simulink model "test"  (R2019b)
settings: Solver=ode45  StartTime=0  StopTime=600  FixedStep=1  MaxStep=1  RelTol=1e-3  EnableMultiTasking=on
values from neighbouring files (symbols this model uses):
  hardware = load_hardware(hardwareN,hardware)    [Simulator.m]
  scenario = Lscenario(scen)    [Simulator.m]    (also in init.m)
  struttura = Lst(ind)    [Simulator.m]    (also in init.m)
undefined symbols (not defined in the file or in its folder): ctrller
settings Model: Creator=Marc Breton  LastModifiedBy=CSLAB
settings SolverCC: InitialStep=0.1
settings DataIOCC: ExternalInput=[t,u]  SaveFormat=Array  SignalLoggingSaveFormat=ModelDataLogs  SaveOutput=off  SignalLogging=off  SaveTime=off  ReturnWorkspaceOutputs=off
settings OptimizationCC: ExpressionDepthLimit=2147483647  InitFltsAndDblsToZero=on  LifeSpan=inf
settings DebuggingCC: SaveWithParameterizedLinksMsg=none  UnderspecifiedInitializationDetection=Classic  MergeDetectMultiDrivingBlocksExec=none  SignalResolutionControl=TryResolveAllWithWarning  SolverPrmCheckMsg=warning  InheritedTsInSrcMsg=none  MultiTaskDSMMsg=warning  MultiTaskCondExecSysMsg=none  FcnCallInpInsideContextMsg=warning  StateNameClashWarn=warning  SFUnexpectedBacktrackingDiag=warning  SFNoUnconditionalDefaultTransitionDiag=warning  SFExecutionAtInitializationDiag=none  ArithmeticOperatorsInVariantConditions=warning
settings HardwareCC: ProdBitPerPointer=32  ProdBitPerSizeT=32  ProdBitPerPtrDiffT=32  ProdLargestAtomicFloat=None  ProdIntDivRoundTo=Undefined  ProdEndianess=Unspecified  ProdWordSize=32  ProdHWDeviceType=32-bit Generic
settings ModelReferenceCC: PropagateSignalLabelsOutOfModel=off
settings SFSimCC: SimUseLocalCustomCode=off  CustomCodeUndefinedFunction=UseInterfaceOnly
settings RTWCC: RTWUseLocalCustomCode=off
settings CodeAppCC: StateflowObjectComments=on
settings GRTTargetCC: TargetFcnLib=ansi_tfl_tmw.mat  TargetLangStandard=C89/C90 (ANSI)  GeneratePreprocessorConditionals=Disable all  CombineOutputUpdateFcns=off  GRTInterface=on
settings ConfigComp: CovMetricSettings=dw  CovHtmlReporting=on  CovSaveCumulativeToWorkspaceVar=on  CovSaveSingleToWorkspaceVar=on  CovExternalEMLEnable=off

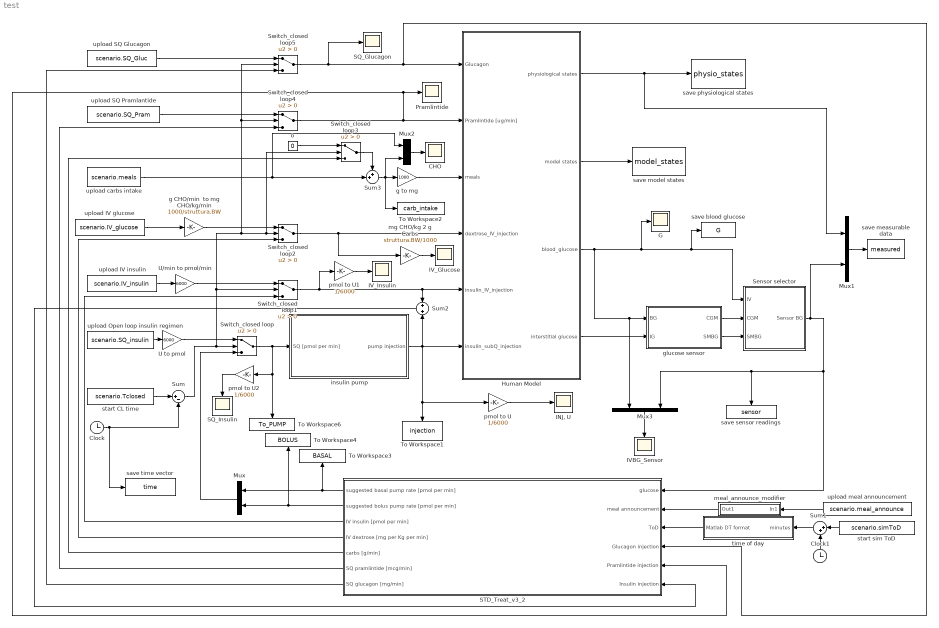
== system test ==
  CHO : Scope
  Clock : Clock
  Clock1 : Clock
  G : Scope
  Human Model : Subsystem
  "INJ, U" : Scope
  IVBG_Sensor : Scope
  IV_Glucose : Scope
  IV_Insulin : Scope
  Mux{,1..3} (4 alike) : Mux  Inputs=2
  Pramlintide : Scope
  SQ_Glucagon : Scope
  SQ_Insulin : Scope
  STD_Treat_v3_2 : Subsystem
  Sensor selector : Subsystem
  Sum : Sum  Inputs=|+-
  Sum1 : Sum  Inputs=|++
  Sum2 : Sum  Inputs=+|+
  Sum3 : Sum  Inputs=++|
  Switch_closed loop{,1..5} (6 alike) : Switch  Criteria=u2 > Threshold
  To Workspace1 : ToWorkspace  VariableName=injection  SaveFormat=Structure  SampleTime=-1
  To Workspace2 : ToWorkspace  VariableName=carb_intake  SaveFormat=Structure  SampleTime=-1
  To Workspace3 : ToWorkspace  VariableName=BASAL  SaveFormat=Structure  SampleTime=-1
  To Workspace4 : ToWorkspace  VariableName=BOLUS  SaveFormat=Structure  SampleTime=-1
  To Workspace6 : ToWorkspace  VariableName=To_PUMP  SaveFormat=Structure  SampleTime=-1
  U to pmol : Gain  Gain=6000
  U/min to pmol/min : Gain  Gain=6000
  g CHO/min  to mg CHO/kg/min : Gain  Gain=1000/struttura.BW
  g to mg : Gain  Gain=1000
  glucose sensor : Subsystem
  insulin pump : Subsystem
  meal_announce_modifier : Subsystem
  mg CHO/kg 2 g Carbs : Gain  Gain=struttura.BW/1000
  o : Constant  Value=0
  pmol to U : Gain  Gain=1/6000
  pmol to U1 : Gain  Gain=1/6000
  pmol to U2 : Gain  Gain=1/6000
  save blood glucose : ToWorkspace  VariableName=G  SaveFormat=Structure  SampleTime=-1
  save measurable data : ToWorkspace  VariableName=measured  SaveFormat=Structure  SampleTime=-1
  save model states : ToWorkspace  VariableName=model_states  SaveFormat=Structure With Time  SampleTime=-1
  save physiological states : ToWorkspace  VariableName=physio_states  SaveFormat=Structure With Time  SampleTime=-1
  save sensor readings : ToWorkspace  VariableName=sensor  SaveFormat=Structure  SampleTime=-1
  save time vector : ToWorkspace  VariableName=time  SaveFormat=Structure  SampleTime=-1
  start CL time : Constant  Value=scenario.Tclosed
  start sim ToD : Constant  Value=scenario.simToD
  time of day : Subsystem
  "upload IV glucose " : FromWorkspace  VariableName=scenario.IV_glucose  SampleTime=0
  upload IV insulin : FromWorkspace  VariableName=scenario.IV_insulin  SampleTime=0
  upload Open loop insulin regimen : FromWorkspace  VariableName=scenario.SQ_insulin  SampleTime=0
  upload SQ Glucagon : FromWorkspace  VariableName=scenario.SQ_Gluc  SampleTime=0
  upload SQ Pramlantide : FromWorkspace  VariableName=scenario.SQ_Pram  SampleTime=0
  upload carbs intake : FromWorkspace  VariableName=scenario.meals  SampleTime=0
  upload meal announcement : FromWorkspace  VariableName=scenario.meal_announce  SampleTime=0
  wires:
  Clock/1 -> Sum/2, save time vector/1
  upload carbs intake/1 -> Mux2/1, Sum3/2
  upload Open loop insulin regimen/1 -> U to pmol/1
  start CL time/1 -> Sum/1
  Sum/1 -> Switch_closed loop/2, Switch_closed loop1/2, Switch_closed loop2/2, Switch_closed loop3/2, Switch_closed loop4/2, Switch_closed loop5/2
  U to pmol/1 -> Switch_closed loop/1
  insulin pump/1(pump injection) -> Human Model/6(insulin_subQ_injection), Sum2/2, To Workspace1/1, pmol to U/1
  Switch_closed loop/1 -> To Workspace6/1, pmol to U2/1, insulin pump/1(SQ [pmol per min])
  STD_Treat_v3_2/1(suggested basal pump rate [pmol per min]) -> Mux/1, To Workspace3/1
  Mux/1 -> Switch_closed loop/3
  start sim ToD/1 -> Sum1/1
  Sum1/1 -> time of day/1(minutes)
  Human Model/1(physiological states) -> save physiological states/1, Mux1/1
  Human Model/2(model states) -> save model states/1
  Human Model/4(interstitial glucose) -> glucose sensor/2(IG)
  "upload IV glucose "/1 -> g CHO/min  to mg CHO/kg/min/1
  upload IV insulin/1 -> U/min to pmol/min/1
  glucose sensor/1(CGM) -> Sensor selector/2(CGM)
  Sensor selector/1(Sensor BG) -> Mux1/2, Mux3/2, save sensor readings/1, STD_Treat_v3_2/1(glucose)
  Sum2/1 -> STD_Treat_v3_2/6(Insulin injection)
  Mux1/1 -> save measurable data/1
  U/min to pmol/min/1 -> Switch_closed loop1/1
  g CHO/min  to mg CHO/kg/min/1 -> Switch_closed loop2/1
  Switch_closed loop1/1 -> Sum2/1, Human Model/5(insulin_IV_injection), pmol to U1/1
  STD_Treat_v3_2/3(IV insulin [pmol per min]) -> Switch_closed loop1/3
  Sum3/1 -> g to mg/1, To Workspace2/1, Mux2/2
  Switch_closed loop3/1 -> Sum3/1
  o/1 -> Switch_closed loop3/1
  glucose sensor/2(SMBG) -> Sensor selector/3(SMBG)
  Clock1/1 -> Sum1/2
  STD_Treat_v3_2/2(suggested bolus pump rate [pmol per min]) -> Mux/2, To Workspace4/1
  STD_Treat_v3_2/4(IV dextrose [mg per Kg per min]) -> Switch_closed loop2/3
  STD_Treat_v3_2/5(carbs [g/min]) -> Switch_closed loop3/3
  time of day/1(Matlab DT format) -> STD_Treat_v3_2/3(ToD)
  pmol to U/1 -> "INJ, U"/1
  upload SQ Pramlantide/1 -> Switch_closed loop4/1
  STD_Treat_v3_2/6(SQ pramlintide [mcg/min]) -> Switch_closed loop4/3
  Switch_closed loop4/1 -> Human Model/2(Pramlintide [ug/min]), STD_Treat_v3_2/5(Pramlintide injection), Pramlintide/1
  Mux2/1 -> CHO/1
  Switch_closed loop5/1 -> Human Model/1(Glucagon), STD_Treat_v3_2/4(Glucagon injection), SQ_Glucagon/1
  STD_Treat_v3_2/7(SQ glucagon [mg/min]) -> Switch_closed loop5/3
  upload SQ Glucagon/1 -> Switch_closed loop5/1
  g to mg/1 -> Human Model/3(meals)
  Switch_closed loop2/1 -> Human Model/4(dextrose_IV_injection), mg CHO/kg 2 g Carbs/1
  meal_announce_modifier/1(Out1) -> STD_Treat_v3_2/2(meal announcement)
  upload meal announcement/1 -> meal_announce_modifier/1(In1)
  Human Model/3(blood_glucose) -> Mux3/1, glucose sensor/1(BG), G/1, save blood glucose/1, Sensor selector/1(IV)
  Mux3/1 -> IVBG_Sensor/1
  pmol to U1/1 -> IV_Insulin/1
  mg CHO/kg 2 g Carbs/1 -> IV_Glucose/1
  pmol to U2/1 -> SQ_Insulin/1

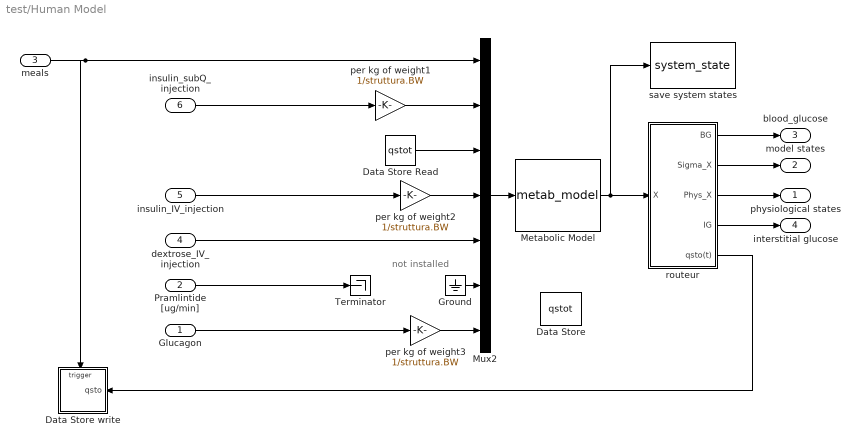
== system test/Human Model ==
  note: not
      | installed
  Glucagon : Inport
  Pramlintide [ug/min] : Inport  Port=2
  meals : Inport  Port=3
  dextrose_IV_injection : Inport  Port=4
  insulin_IV_injection : Inport  Port=5
  insulin_subQ_injection : Inport  Port=6
  Data Store : DataStoreMemory  DataStoreName=qstot  ShowAdditionalParam=off
  Data Store Read : DataStoreRead  DataStoreName=qstot
  Data Store write : Subsystem  TreatAsAtomicUnit=on
  Ground : Ground
  Metabolic Model : S-Function  FunctionName=metab_model  Parameters=struttura  SFunctionDeploymentMode=off  EnableBusSupport=off
  Mux2 : Mux  Inputs=7
  Terminator : Terminator
  per kg of weight1 : Gain  Gain=1/struttura.BW
  per kg of weight2 : Gain  Gain=1/struttura.BW
  per kg of weight3 : Gain  Gain=1/struttura.BW
  routeur : Subsystem
  save system states : ToWorkspace  VariableName=system_state  SaveFormat=Structure With Time  SampleTime=-1
  physiological states : Outport
  model states : Outport  Port=2
  blood_glucose : Outport  Port=3
  interstitial glucose : Outport  Port=4
  wires:
  Metabolic Model/1 -> routeur/1(X), save system states/1
  routeur/3(Phys_X) -> physiological states/1
  routeur/1(BG) -> blood_glucose/1
  insulin_subQ_injection/1 -> per kg of weight1/1
  Mux2/1 -> Metabolic Model/1
  routeur/2(Sigma_X) -> model states/1
  Data Store Read/1 -> Mux2/3
  routeur/4(IG) -> interstitial glucose/1
  per kg of weight1/1 -> Mux2/2
  insulin_IV_injection/1 -> per kg of weight2/1
  dextrose_IV_injection/1 -> Mux2/5
  routeur/5(qsto(t)) -> Data Store write/1(qsto)
  per kg of weight2/1 -> Mux2/4
  meals/1 -> Data Store write/Trigger, Mux2/1
  Pramlintide [ug/min]/1 -> Terminator/1
  Ground/1 -> Mux2/6
  Glucagon/1 -> per kg of weight3/1
  per kg of weight3/1 -> Mux2/7

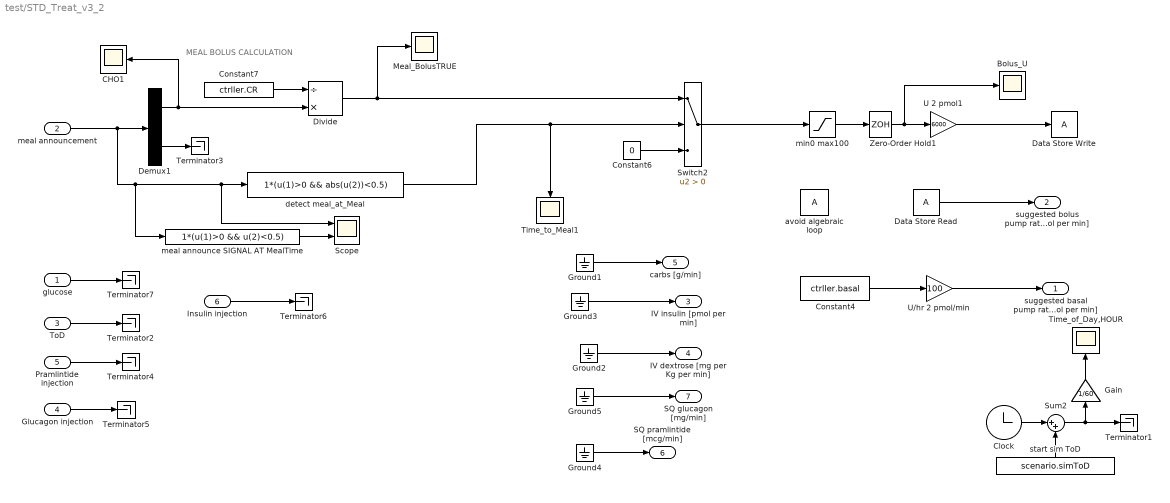
== system test/STD_Treat_v3_2 ==
  note: MEAL BOLUS CALCULATION
  glucose : Inport
  meal announcement : Inport  Port=2
  ToD : Inport  Port=3
  Glucagon injection : Inport  Port=4
  Pramlintide injection : Inport  Port=5
  Insulin injection : Inport  Port=6
  Bolus_U : Scope
  CHO1 : Scope
  Clock : Clock
  Constant4 : Constant  Value=ctrller.basal
  Constant6 : Constant  Value=0
  Constant7 : Constant  Value=ctrller.CR
  Data Store Read : DataStoreRead  SampleTime=0
  Data Store Write : DataStoreWrite
  Demux1 : Demux  Outputs=2
  Divide : Product  Inputs=/*
  Gain : Gain  Gain=1/60
  Ground{1..5} (5 alike) : Ground
  Meal_BolusTRUE : Scope
  Scope : Scope  NumInputPorts=2
  Sum2 : Sum  Inputs=|++
  Switch2 : Switch  Criteria=u2 > Threshold
  Terminator{1..7} (7 alike) : Terminator
  Time_of_Day,HOUR : Scope
  Time_to_Meal1 : Scope
  U 2 pmol1 : Gain  Gain=6000
  U/hr 2 pmol/min : Gain  Gain=100
  Zero-Order Hold1 : ZeroOrderHold
  avoid algebraic loop : DataStoreMemory  ReadBeforeWriteMsg=warning  WriteAfterWriteMsg=warning  WriteAfterReadMsg=warning  ShowAdditionalParam=off
  detect meal_at_Meal : Fcn  Expr=1*(u(1)>0 && abs(u(2))<0.5)
  meal announce SIGNAL AT MealTime : Fcn  Expr=1*(u(1)>0 && u(2)<0.5)  SampleTime=1
  min0 max100 : Saturate  UpperLimit=100  LowerLimit=0
  start sim ToD : Constant  Value=scenario.simToD
  suggested basal pump rate [pmol per min] : Outport
  suggested bolus pump rate [pmol per min] : Outport  Port=2
  IV insulin [pmol per min] : Outport  Port=3
  IV dextrose [mg per Kg per min] : Outport  Port=4
  carbs [g/min] : Outport  Port=5
  SQ pramlintide [mcg/min] : Outport  Port=6
  SQ glucagon [mg/min] : Outport  Port=7
  wires:
  Data Store Read/1 -> suggested bolus pump rate [pmol per min]/1
  U/hr 2 pmol/min/1 -> suggested basal pump rate [pmol per min]/1
  Constant4/1 -> U/hr 2 pmol/min/1
  ToD/1 -> Terminator2/1
  Constant6/1 -> Switch2/3
  detect meal_at_Meal/1 -> Switch2/2, Time_to_Meal1/1
  Constant7/1 -> Divide/1
  Demux1/1 -> Divide/2, CHO1/1
  meal announcement/1 -> Demux1/1, meal announce SIGNAL AT MealTime/1, detect meal_at_Meal/1, Scope/1
  Demux1/2 -> Terminator3/1
  Divide/1 -> Meal_BolusTRUE/1, Switch2/1
  Zero-Order Hold1/1 -> U 2 pmol1/1, Bolus_U/1
  U 2 pmol1/1 -> Data Store Write/1
  min0 max100/1 -> Zero-Order Hold1/1
  Clock/1 -> Sum2/1
  Sum2/1 -> Terminator1/1, Gain/1
  start sim ToD/1 -> Sum2/2
  Gain/1 -> Time_of_Day,HOUR/1
  Ground5/1 -> SQ glucagon [mg/min]/1
  Ground4/1 -> SQ pramlintide [mcg/min]/1
  Pramlintide injection/1 -> Terminator4/1
  Ground2/1 -> IV dextrose [mg per Kg per min]/1
  Glucagon injection/1 -> Terminator5/1
  Ground1/1 -> carbs [g/min]/1
  Ground3/1 -> IV insulin [pmol per min]/1
  meal announce SIGNAL AT MealTime/1 -> Scope/2
  Insulin injection/1 -> Terminator6/1
  glucose/1 -> Terminator7/1
  Switch2/1 -> min0 max100/1

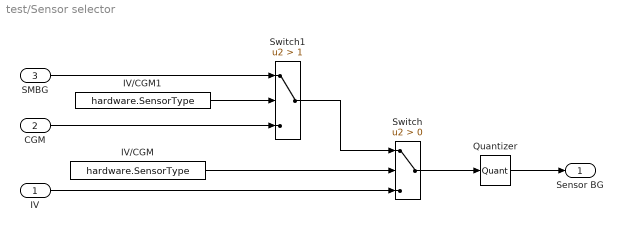
== system test/Sensor selector ==
  IV : Inport
  CGM : Inport  Port=2
  SMBG : Inport  Port=3
  IV/CGM : Constant  Value=hardware.SensorType
  IV/CGM1 : Constant  Value=hardware.SensorType
  Quantizer : Quantizer  QuantizationInterval=1
  Switch : Switch  Criteria=u2 > Threshold
  Switch1 : Switch  Criteria=u2 > Threshold  Threshold=1
  Sensor BG : Outport
  wires:
  IV/1 -> Switch/3
  CGM/1 -> Switch1/3
  Switch1/1 -> Switch/1
  IV/CGM/1 -> Switch/2
  IV/CGM1/1 -> Switch1/2
  SMBG/1 -> Switch1/1
  Quantizer/1 -> Sensor BG/1
  Switch/1 -> Quantizer/1

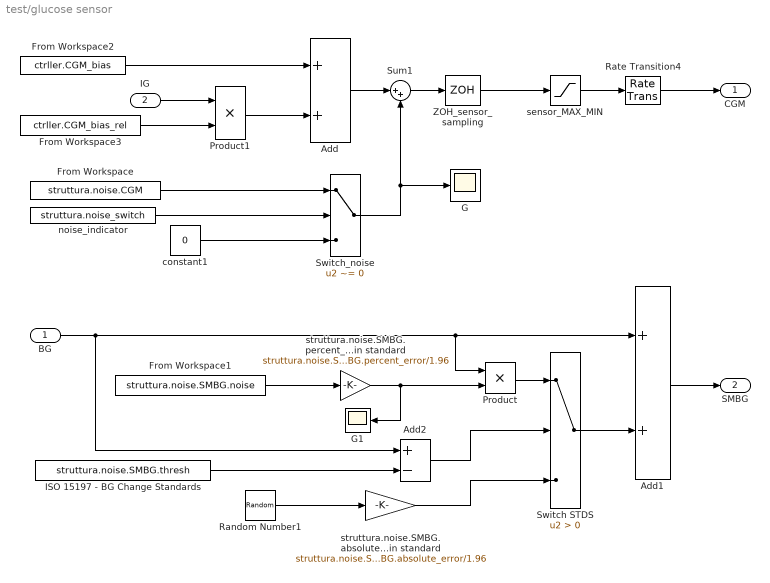
== system test/glucose sensor ==
  BG : Inport
  IG : Inport  Port=2
  Add : Sum
  Add1 : Sum
  Add2 : Sum  Inputs=+-
  From Workspace : FromWorkspace  VariableName=struttura.noise.CGM  SampleTime=0
  From Workspace1 : FromWorkspace  VariableName=struttura.noise.SMBG.noise  SampleTime=0
  From Workspace2 : FromWorkspace  VariableName=ctrller.CGM_bias  SampleTime=0  Interpolate=off  OutputAfterFinalValue=Holding final value
  From Workspace3 : FromWorkspace  VariableName=ctrller.CGM_bias_rel  SampleTime=0  Interpolate=off  OutputAfterFinalValue=Holding final value
  G : Scope
  G1 : Scope
  ISO 15197 - BG Change Standards : Constant  Value=struttura.noise.SMBG.thresh
  Product : Product  RndMeth=Zero
  Product1 : Product  RndMeth=Zero
  Random Number1 : RandomNumber  Variance=0.2  Seed=1  SampleTime=1
  Rate Transition4 : RateTransition  InitialCondition=struttura.x0(4)/struttura.Vg  OutPortSampleTime=1
  Sum1 : Sum  Inputs=|++
  Switch STDS : Switch  Criteria=u2 > Threshold
  Switch_noise : Switch  Criteria=u2 ~= 0  Threshold=1440
  ZOH_sensor_sampling : ZeroOrderHold  SampleTime=hardware.sensor_sampling
  constant1 : Constant  Value=0
  noise_indicator : Constant  Value=struttura.noise_switch
  sensor_MAX_MIN : Saturate  UpperLimit=hardware.sensor_max  LowerLimit=hardware.sensor_min
  struttura.noise.SMBG.absolute_error/1.96 95% of values to fall within standard : Gain  Gain=struttura.noise.SMBG.absolute_error/1.96
  struttura.noise.SMBG.percent_error/1.96 95% of values to fall within standard : Gain  Gain=struttura.noise.SMBG.percent_error/1.96
  CGM : Outport
  SMBG : Outport  Port=2
  wires:
  Sum1/1 -> ZOH_sensor_sampling/1
  ZOH_sensor_sampling/1 -> sensor_MAX_MIN/1
  sensor_MAX_MIN/1 -> Rate Transition4/1
  From Workspace/1 -> Switch_noise/1
  noise_indicator/1 -> Switch_noise/2
  constant1/1 -> Switch_noise/3
  Switch_noise/1 -> Sum1/2, G/1
  IG/1 -> Product1/1
  From Workspace2/1 -> Add/1
  Product1/1 -> Add/2
  Add/1 -> Sum1/1
  Rate Transition4/1 -> CGM/1
  From Workspace1/1 -> struttura.noise.SMBG.percent_error/1.96 95% of values to fall within standard/1
  BG/1 -> Add2/1, Add1/1, Product/1
  ISO 15197 - BG Change Standards/1 -> Add2/2
  struttura.noise.SMBG.percent_error/1.96 95% of values to fall within standard/1 -> Product/2, G1/1
  Product/1 -> Switch STDS/1
  Switch STDS/1 -> Add1/2
  Add2/1 -> Switch STDS/2
  Random Number1/1 -> struttura.noise.SMBG.absolute_error/1.96 95% of values to fall within standard/1
  struttura.noise.SMBG.absolute_error/1.96 95% of values to fall within standard/1 -> Switch STDS/3
  Add1/1 -> SMBG/1
  From Workspace3/1 -> Product1/2

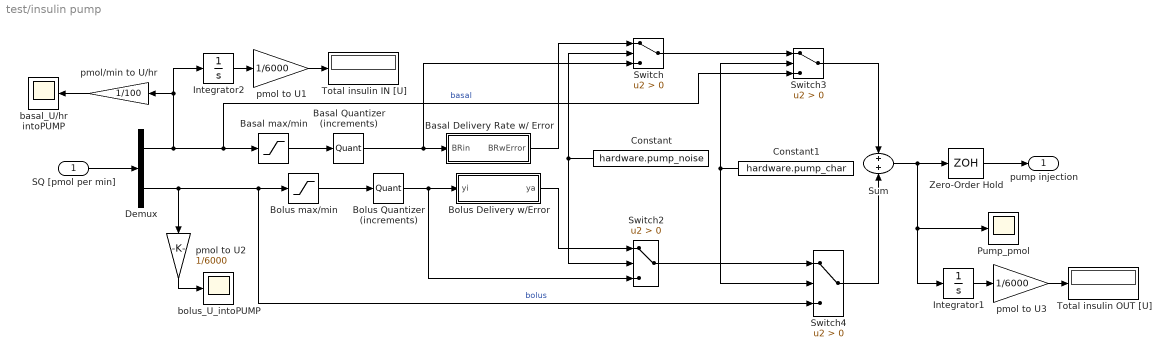
== system test/insulin pump ==
  SQ [pmol per min] : Inport
  Basal Delivery Rate w/ Error : Subsystem
  Basal Quantizer (increments) : Quantizer  QuantizationInterval=hardware.pump_basal_inc
  Basal max/min : Saturate  UpperLimit=hardware.pump_basal_max  LowerLimit=hardware.pump_basal_min
  Bolus Delivery w/Error : Subsystem
  Bolus Quantizer (increments) : Quantizer  QuantizationInterval=hardware.pump_bolus_inc
  Bolus max/min : Saturate  UpperLimit=hardware.pump_bolus_max  LowerLimit=0
  Constant : Constant  Value=hardware.pump_noise
  Constant1 : Constant  Value=hardware.pump_char
  Demux : Demux  Outputs=2
  Integrator1 : Integrator
  Integrator2 : Integrator
  Pump_pmol : Scope
  Sum : Sum  Inputs=+|+
  Switch{,2..4} (4 alike) : Switch  Criteria=u2 > Threshold
  Total insulin IN [U] : Display
  Total insulin OUT [U] : Display
  Zero-Order Hold : ZeroOrderHold
  basal_U/hr intoPUMP : Scope
  bolus_U_intoPUMP : Scope
  pmol to U1 : Gain  Gain=1/6000
  pmol to U2 : Gain  Gain=1/6000
  pmol to U3 : Gain  Gain=1/6000
  pmol/min to U/hr : Gain  Gain=1/100
  pump injection : Outport
  wires:
  Zero-Order Hold/1 -> pump injection/1
  pmol to U1/1 -> Total insulin IN [U]/1
  Integrator2/1 -> pmol to U1/1
  Bolus max/min/1 -> Bolus Quantizer (increments)/1
  SQ [pmol per min]/1 -> Demux/1
  Sum/1 -> Zero-Order Hold/1, Pump_pmol/1, Integrator1/1
  Demux/1 -> Basal max/min/1, Switch3/3, Integrator2/1, pmol/min to U/hr/1  "basal"
  Basal max/min/1 -> Basal Quantizer (increments)/1
  Demux/2 -> Bolus max/min/1, Switch4/3, pmol to U2/1  "bolus"
  Bolus Quantizer (increments)/1 -> Switch2/3, Bolus Delivery w/Error/1(yi)
  Basal Quantizer (increments)/1 -> Switch/3, Basal Delivery Rate w/ Error/1(BRin)
  Basal Delivery Rate w/ Error/1(BRwError) -> Switch/1
  Constant/1 -> Switch2/2, Switch/2
  Bolus Delivery w/Error/1(ya) -> Switch2/1
  Switch2/1 -> Switch4/1
  Switch/1 -> Switch3/1
  Constant1/1 -> Switch4/2, Switch3/2
  Switch3/1 -> Sum/1
  Switch4/1 -> Sum/2
  pmol to U2/1 -> bolus_U_intoPUMP/1
  pmol/min to U/hr/1 -> basal_U/hr intoPUMP/1
  pmol to U3/1 -> Total insulin OUT [U]/1
  Integrator1/1 -> pmol to U3/1

== system test/meal_announce_modifier ==
  In1 : Inport
  Demux : Demux  Outputs=2
  From Workspace : FromWorkspace  VariableName=ctrller.meal_announce_modifier  SampleTime=0  Interpolate=off  OutputAfterFinalValue=Holding final value
  Mux : Mux  Inputs=2
  Product : Product  RndMeth=Zero
  Out1 : Outport
  wires:
  Product/1 -> Mux/1
  From Workspace/1 -> Product/1
  Demux/1 -> Product/2
  Demux/2 -> Mux/2
  In1/1 -> Demux/1
  Mux/1 -> Out1/1

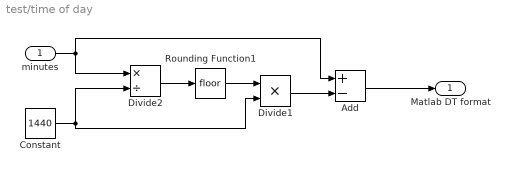
== system test/time of day ==
  minutes : Inport
  Add : Sum  Inputs=+-
  Constant : Constant  Value=1440
  Divide1 : Product  Inputs=**
  Divide2 : Product  Inputs=*/
  Rounding Function1 : Rounding
  Matlab DT format : Outport
  wires:
  minutes/1 -> Divide2/1, Add/1
  Constant/1 -> Divide2/2, Divide1/2
  Divide2/1 -> Rounding Function1/1
  Rounding Function1/1 -> Divide1/1
  Divide1/1 -> Add/2
  Add/1 -> Matlab DT format/1

== system test/Human Model/Data Store write ==
  qsto : Inport  LatchByDelayingOutsideSignal=on
  Trigger : TriggerPort  VariantControl=(inherit)
  Data Store Write : DataStoreWrite  DataStoreName=qstot
  wires:
  qsto/1 -> Data Store Write/1

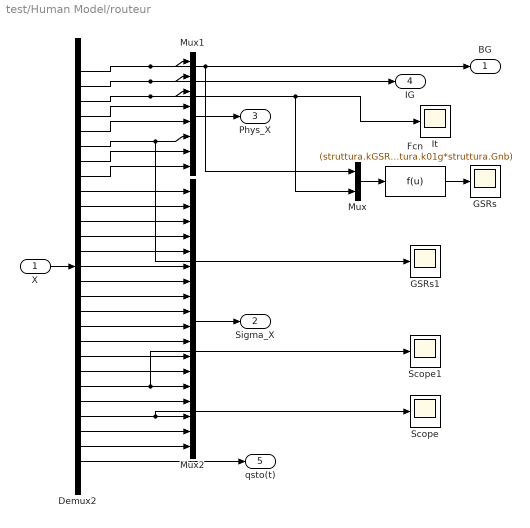
== system test/Human Model/routeur ==
  X : Inport
  Demux2 : Demux  Outputs=27
  Fcn : Fcn  Expr=(struttura.kGSRs*(struttura.Gth-(u(1)))/((u(2)-struttura.Ith)+1)+struttura.k01g*struttura.Gnb)
  GSRs : Scope
  GSRs1 : Scope
  It : Scope
  Mux : Mux  Inputs=2
  Mux1 : Mux  Inputs=8
  Mux2 : Mux  Inputs=18
  Scope : Scope
  Scope1 : Scope
  BG : Outport
  Sigma_X : Outport  Port=2
  Phys_X : Outport  Port=3
  IG : Outport  Port=4
  qsto(t) : Outport  Port=5
  wires:
  X/1 -> Demux2/1
  Mux1/1 -> Phys_X/1
  Demux2/1 -> Mux1/1, BG/1, Mux/1
  Demux2/2 -> Mux1/2, IG/1
  Demux2/3 -> Mux1/3, It/1, Mux/2
  Demux2/4 -> Mux1/4
  Demux2/5 -> Mux1/5
  Demux2/6 -> Mux1/6, GSRs1/1
  Demux2/7 -> Mux1/7
  Demux2/8 -> Mux1/8
  Demux2/9 -> Mux2/1
  Demux2/10 -> Mux2/2
  Demux2/11 -> Mux2/3
  Demux2/12 -> Mux2/4
  Demux2/13 -> Mux2/5
  Demux2/14 -> Mux2/6
  Demux2/15 -> Mux2/7
  Demux2/16 -> Mux2/8
  Demux2/17 -> Mux2/9
  Demux2/18 -> Mux2/10
  Demux2/19 -> Mux2/11
  Mux2/1 -> Sigma_X/1
  Mux/1 -> Fcn/1
  Fcn/1 -> GSRs/1
  Demux2/27 -> qsto(t)/1
  Demux2/20 -> Mux2/12
  Demux2/21 -> Mux2/13
  Demux2/22 -> Scope1/1, Mux2/14
  Demux2/23 -> Mux2/15
  Demux2/24 -> Mux2/16, Scope/1
  Demux2/25 -> Mux2/17
  Demux2/26 -> Mux2/18

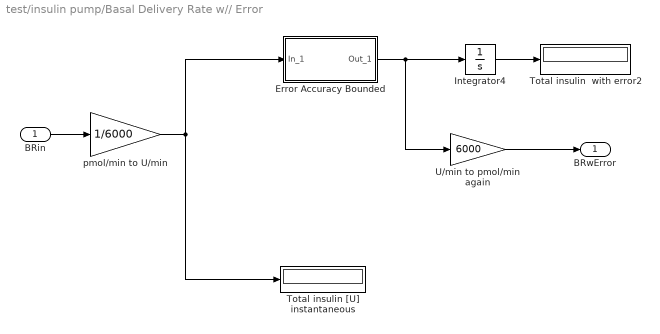
== system test/insulin pump/Basal Delivery Rate w// Error ==
  BRin : Inport
  Error Accuracy Bounded : Subsystem
  Integrator4 : Integrator
  Total insulin  with error2 : Display
  Total insulin [U] instantaneous : Display
  U/min to pmol/min again : Gain  Gain=6000
  pmol/min to U/min : Gain  Gain=1/6000
  BRwError : Outport
  wires:
  Integrator4/1 -> Total insulin  with error2/1
  Error Accuracy Bounded/1(Out_1) -> Integrator4/1, U/min to pmol/min again/1
  U/min to pmol/min again/1 -> BRwError/1
  pmol/min to U/min/1 -> Error Accuracy Bounded/1(In_1), Total insulin [U] instantaneous/1
  BRin/1 -> pmol/min to U/min/1

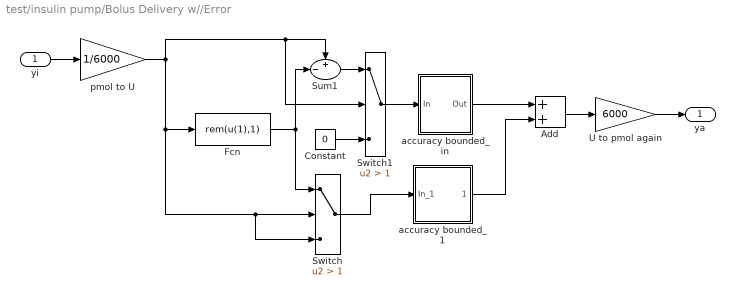
== system test/insulin pump/Bolus Delivery w//Error ==
  yi : Inport
  Add : Sum
  Constant : Constant  Value=0
  Fcn : Fcn  Expr=rem(u(1),1)
  Sum1 : Sum  Inputs=+-|
  Switch : Switch  Criteria=u2 > Threshold  Threshold=1
  Switch1 : Switch  Criteria=u2 > Threshold  Threshold=1
  U to pmol again : Gain  Gain=6000
  accuracy bounded_1 : Subsystem
  accuracy bounded_in : Subsystem
  pmol to U : Gain  Gain=1/6000
  ya : Outport
  wires:
  Switch1/1 -> accuracy bounded_in/1(In)
  Constant/1 -> Switch1/3
  Sum1/1 -> Switch1/1
  Switch/1 -> accuracy bounded_1/1(In_1)
  Fcn/1 -> Sum1/2, Switch/1
  accuracy bounded_1/1(Out_1) -> Add/2
  accuracy bounded_in/1(Out) -> Add/1
  Add/1 -> U to pmol again/1
  U to pmol again/1 -> ya/1
  pmol to U/1 -> Switch1/2, Sum1/1, Switch/3, Switch/2, Fcn/1
  yi/1 -> pmol to U/1

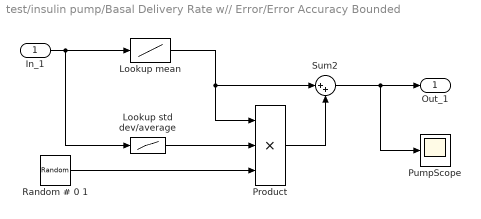
== system test/insulin pump/Basal Delivery Rate w// Error/Error Accuracy Bounded ==
  In_1 : Inport
  Lookup mean : Lookup  InputValues=hardware.pump_accuracy_bolus_amount  Table=hardware.pump_bolus_mean
  Lookup std dev/average : Lookup  InputValues=hardware.pump_accuracy_bolus_amount  Table=hardware.pump_bolus_std2r
  Product : Product  Inputs=3  RndMeth=Zero
  PumpScope : Scope
  "Random # 0 1 " : RandomNumber  SampleTime=1
  Sum2 : Sum  Inputs=|++
  Out_1 : Outport
  wires:
  In_1/1 -> Lookup std dev/average/1, Lookup mean/1
  "Random # 0 1 "/1 -> Product/3
  Lookup std dev/average/1 -> Product/2
  Product/1 -> Sum2/2
  Sum2/1 -> Out_1/1, PumpScope/1
  Lookup mean/1 -> Sum2/1, Product/1

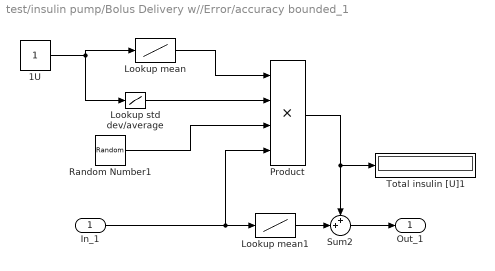
== system test/insulin pump/Bolus Delivery w//Error/accuracy bounded_1 ==
  In_1 : Inport
  1U : Constant
  Lookup mean : Lookup  InputValues=hardware.pump_accuracy_bolus_amount  Table=hardware.pump_bolus_mean  LookUpMeth=Interpolation-Use End Values
  Lookup mean1 : Lookup  InputValues=hardware.pump_accuracy_bolus_amount  Table=hardware.pump_bolus_mean
  Lookup std dev/average : Lookup  InputValues=hardware.pump_accuracy_bolus_amount  Table=hardware.pump_bolus_std2r  LookUpMeth=Interpolation-Use End Values
  Product : Product  Inputs=4  RndMeth=Zero
  Random Number1 : RandomNumber  SampleTime=1
  Sum2 : Sum  Inputs=++|
  Total insulin [U]1 : Display
  Out_1 : Outport
  wires:
  Product/1 -> Total insulin [U]1/1, Sum2/1
  Lookup mean1/1 -> Sum2/2
  In_1/1 -> Lookup mean1/1, Product/4
  1U/1 -> Lookup std dev/average/1, Lookup mean/1
  Sum2/1 -> Out_1/1
  Random Number1/1 -> Product/3
  Lookup std dev/average/1 -> Product/2
  Lookup mean/1 -> Product/1

== system test/insulin pump/Bolus Delivery w//Error/accuracy bounded_in ==
  In : Inport
  Lookup mean : Lookup  InputValues=hardware.pump_accuracy_bolus_amount  Table=hardware.pump_bolus_mean
  Lookup std dev/average : Lookup  InputValues=hardware.pump_accuracy_bolus_amount  Table=hardware.pump_bolus_std2r  LookUpMeth=Interpolation-Use End Values
  Product : Product  Inputs=3  RndMeth=Zero
  Random Number1 : RandomNumber  SampleTime=1
  Sum2 : Sum  Inputs=|++
  Out : Outport
  wires:
  Sum2/1 -> Out/1
  In/1 -> Lookup mean/1, Lookup std dev/average/1
  Product/1 -> Sum2/2
  Lookup mean/1 -> Sum2/1, Product/1
  Random Number1/1 -> Product/3
  Lookup std dev/average/1 -> Product/2
